simulink model "Simulink_lab2"  (R2019a)
settings: Solver=FixedStepAuto  StartTime=0.0  StopTime=10.0  FixedStep=1e-3  RelTol=1e-3
settings Model: Creator=T.S  LastModifiedBy=T.S

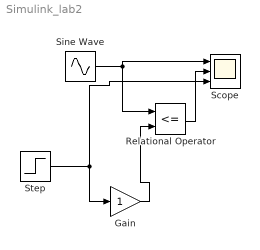
== system Simulink_lab2 ==
  Gain : Gain
  Relational Operator : RelationalOperator  Operator=<=  OutDataTypeStr=boolean  RndMeth=Simplest
  Scope : Scope  NumInputPorts=3
  Sine Wave : Sin  Frequency=2*pi*1  SampleTime=0
  Step : Step  Time=2  SampleTime=0
  wires:
  Sine Wave/1 -> Relational Operator/1, Scope/1
  Relational Operator/1 -> Scope/2
  Step/1 -> Gain/1, Scope/3
  Gain/1 -> Relational Operator/2
